simulink model "state_estimator"  (Simulink 9.1)
settings: Solver=VariableStepAuto  StartTime=0.0  StopTime=10.0  RelTol=1e-3
values from neighbouring files (symbols this model uses):
  Estimator =     [data_set.mat]
  g = 9.81    [data_set.mat]
  init =     [data_set.mat]
  Sensors =     [data_set.mat]
  Ts = 0.005    [data_set.mat]
undefined symbols (not defined in the file or in its folder): DiscIntNeverNeededParam, Discrete, Time
libraries: F_Line_block x281, simulink x27, ctrlSharedLib x3, sharedtransform x3, sharedutil x1
(part 1 of 2)
settings Model: LogicAnalyzerSignalOrdering=8909f14e-64a4-4a01-80b1-dba654a4ac6a  Creator=dongw  LastModifiedBy=dongw
settings DataIOCC: SaveFormat=Dataset
settings OptimizationCC: LifeSpan=auto
settings DebuggingCC: UnderspecifiedInitializationDetection=Simplified  MergeDetectMultiDrivingBlocksExec=error  SFUnexpectedBacktrackingDiag=error  SFNoUnconditionalDefaultTransitionDiag=error  SFExecutionAtInitializationDiag=warning
settings HardwareCC: ProdBitPerPointer=64  ProdBitPerSizeT=64  ProdBitPerPtrDiffT=64  ProdLargestAtomicFloat=Float  ProdIntDivRoundTo=Zero  ProdEndianess=LittleEndian  ProdWordSize=64  ProdHWDeviceType=Intel->x86-64 (Windows64)
settings ModelReferenceCC: PropagateSignalLabelsOutOfModel=on
settings CodeAppCC: StateflowObjectComments=off
settings GRTTargetCC: TargetLangStandard=C99 (ISO)  CombineOutputUpdateFcns=on  GRTInterface=off
settings ConfigComp: CovMetricSettings=dwe  CovHtmlReporting=off  CovSaveCumulativeToWorkspaceVar=off  CovSaveSingleToWorkspaceVar=off  CovExternalEMLEnable=on

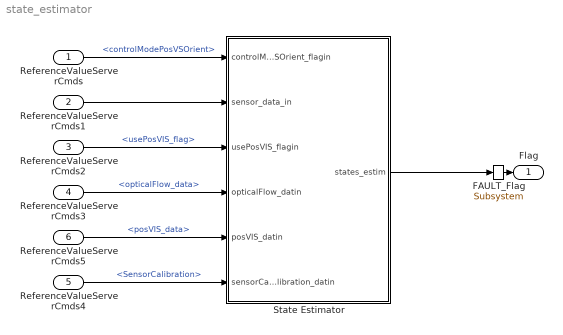
== system state_estimator ==
  ReferenceValueServerCmds : Inport  OutDataTypeStr=Bus: CommandBus
  ReferenceValueServerCmds1 : Inport  Port=2  OutDataTypeStr=Bus: CommandBus
  ReferenceValueServerCmds2 : Inport  Port=3  OutDataTypeStr=Bus: CommandBus
  ReferenceValueServerCmds3 : Inport  Port=4  OutDataTypeStr=Bus: CommandBus
  ReferenceValueServerCmds4 : Inport  Port=5  OutDataTypeStr=Bus: CommandBus
  ReferenceValueServerCmds5 : Inport  Port=6  OutDataTypeStr=Bus: CommandBus
  State Estimator : Subsystem
  Flag : Outport
  FAULT_Flag : F_Line_block/Subsystem
  wires:
  ReferenceValueServerCmds5/1 -> State Estimator/5(posVIS_datin)  "<posVIS_data>"
  State Estimator/1(states_estim) -> FAULT_Flag/1
  FAULT_Flag/1 -> Flag/1
  ReferenceValueServerCmds4/1 -> State Estimator/6(sensorCalibration_datin)  "<SensorCalibration>"
  ReferenceValueServerCmds2/1 -> State Estimator/3(usePosVIS_flagin)  "<usePosVIS_flag>"
  ReferenceValueServerCmds/1 -> State Estimator/1(controlModePosVSOrient_flagin)  "<controlModePosVSOrient>"
  ReferenceValueServerCmds3/1 -> State Estimator/4(opticalFlow_datin)  "<opticalFlow_data>"
  ReferenceValueServerCmds1/1 -> State Estimator/2(sensor_data_in)

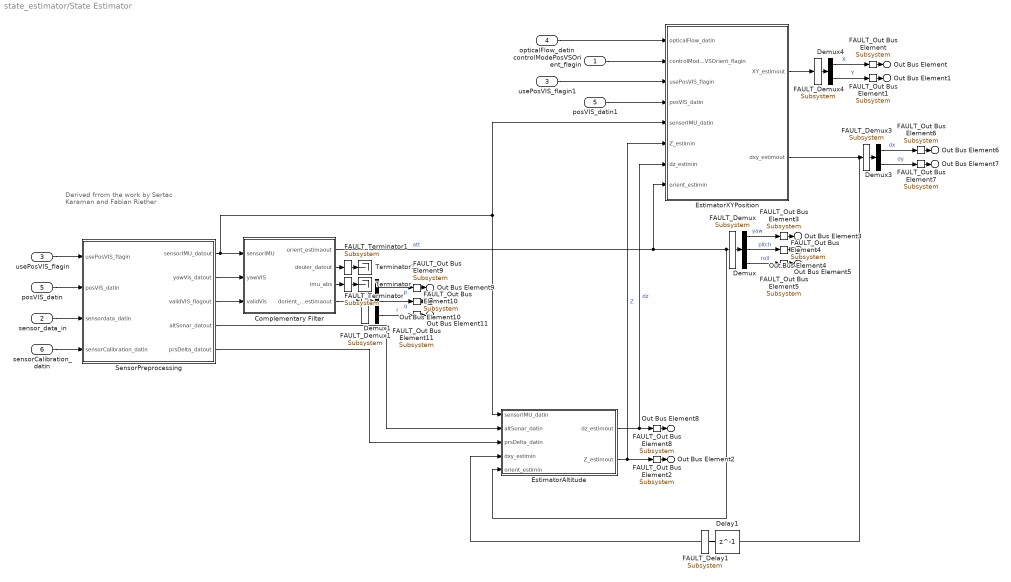
== system state_estimator/State Estimator ==
  note: Derived frrom the work by Sertac
      | Karaman and Fabian Riether
  controlModePosVSOrient_flagin : Inport  OutDataTypeStr=boolean
  sensor_data_in : Inport  Port=2
  usePosVIS_flagin : Inport  Port=3
  opticalFlow_datin : Inport  Port=4
  posVIS_datin : Inport  Port=5
  sensorCalibration_datin : Inport  Port=6
  Complementary Filter : Subsystem
  Delay1 : Delay  DelayLength=1  InitialCondition=0
  FAULT_Delay1 : F_Line_block/Subsystem
  Demux : Demux  Outputs=3
  FAULT_Demux{,1,3..4} (4 alike) : F_Line_block/Subsystem
  Demux1 : Demux  Outputs=3
  Demux3 : Demux  Outputs=2
  Demux4 : Demux  Outputs=2
  EstimatorAltitude : Subsystem
  EstimatorXYPosition : Subsystem
  SensorPreprocessing : Subsystem
  Terminator : Terminator
  FAULT_Terminator : F_Line_block/Subsystem
  Terminator1 : Terminator
  FAULT_Terminator1 : F_Line_block/Subsystem
  posVIS_datin1 : InportShadow  Port=5
  usePosVIS_flagin1 : InportShadow  Port=3
  Out Bus Element : Outport  PortName=states_estim  Element=X
  FAULT_Out Bus Element{,1..11} (12 alike) : F_Line_block/Subsystem
  Out Bus Element1 : Outport  PortName=states_estim  Element=Y
  Out Bus Element2 : Outport  PortName=states_estim  Element=Z
  Out Bus Element3 : Outport  PortName=states_estim  Element=yaw
  Out Bus Element4 : Outport  PortName=states_estim  Element=pitch
  Out Bus Element5 : Outport  PortName=states_estim  Element=roll
  Out Bus Element6 : Outport  PortName=states_estim  Element=dx
  Out Bus Element7 : Outport  PortName=states_estim  Element=dy
  Out Bus Element8 : Outport  PortName=states_estim  Element=dz
  Out Bus Element9 : Outport  PortName=states_estim  Element=p
  Out Bus Element10 : Outport  PortName=states_estim  Element=q
  Out Bus Element11 : Outport  PortName=states_estim  Element=r
  wires:
  EstimatorXYPosition/2(dxy_estimout) -> FAULT_Delay1/1, FAULT_Demux3/1
  ?FAULT_dxy_estimout_		DstPort			1/1 -> ?dxy_estimout/dstport			1
  ?FAULT_KalmanFilter_posxy/1 -> ?KalmanFilter_posxy/1
  ?FAULT_Mux1_6/1 -> ?Mux1/6
  ?FAULT_Product_2/1 -> ?Product/2
  FAULT_Delay1/1 -> Delay1/1
  FAULT_Demux3/1 -> Demux3/1
  posVIS_datin/1 -> SensorPreprocessing/2(posVIS_datin)
  Demux1/3 -> FAULT_Out Bus Element11/1  "r"
  FAULT_Out Bus Element11/1 -> Out Bus Element11/1
  Demux/3 -> FAULT_Out Bus Element5/1  "roll"
  FAULT_Out Bus Element5/1 -> Out Bus Element5/1
  Demux4/2 -> FAULT_Out Bus Element1/1  "Y"
  FAULT_Out Bus Element1/1 -> Out Bus Element1/1
  EstimatorXYPosition/1(XY_estimout) -> FAULT_Demux4/1
  FAULT_Demux4/1 -> Demux4/1
  Complementary Filter/2(deuler_datout) -> FAULT_Terminator1/1
  FAULT_Terminator1/1 -> Terminator1/1
  Complementary Filter/4(dorient_estimaout) -> FAULT_Demux1/1
  FAULT_Demux1/1 -> Demux1/1
  SensorPreprocessing/3(validVIS_flagout) -> Complementary Filter/3(validVis)
  sensor_data_in/1 -> SensorPreprocessing/3(sensordata_datin)
  opticalFlow_datin/1 -> EstimatorXYPosition/1(opticalFlow_datin)
  Demux4/1 -> FAULT_Out Bus Element/1  "X"
  FAULT_Out Bus Element/1 -> Out Bus Element/1
  SensorPreprocessing/1(sensorIMU_datout) -> Complementary Filter/1(sensorIMU), EstimatorAltitude/1(sensorIMU_datin), EstimatorXYPosition/5(sensorIMU_datin)
  SensorPreprocessing/5(prsDelta_datout) -> EstimatorAltitude/3(prsDelta_datin)
  Demux3/2 -> FAULT_Out Bus Element7/1  "dy"
  ?FAULT_dxy_estimout_		DstPort			1/1 -> ?dxy_estimout/dstport			1
  ?FAULT_KalmanFilter_posxy/1 -> ?KalmanFilter_posxy/1
  ?FAULT_Mux1_6/1 -> ?Mux1/6
  FAULT_Out Bus Element7/1 -> Out Bus Element7/1
  SensorPreprocessing/2(yawVis_datout) -> Complementary Filter/2(yawVIS)
  SensorPreprocessing/4(altSonar_datout) -> EstimatorAltitude/2(altSonar_datin)
  usePosVIS_flagin/1 -> SensorPreprocessing/1(usePosVIS_flagin)
  EstimatorAltitude/1(dz_estimout) -> FAULT_Out Bus Element8/1, EstimatorXYPosition/7(dz_estimin)  "dz"
  FAULT_Out Bus Element8/1 -> Out Bus Element8/1
  ?FAULT_KalmanFilter_posxy/1 -> ?KalmanFilter_posxy/1
  EstimatorAltitude/2(Z_estimout) -> FAULT_Out Bus Element2/1, EstimatorXYPosition/6(Z_estimin)  "Z"
  FAULT_Out Bus Element2/1 -> Out Bus Element2/1
  ?FAULT_KalmanFilter_posxy/1 -> ?KalmanFilter_posxy/1
  Demux1/1 -> FAULT_Out Bus Element9/1  "p"
  FAULT_Out Bus Element9/1 -> Out Bus Element9/1
  Demux3/1 -> FAULT_Out Bus Element6/1  "dx"
  FAULT_Out Bus Element6/1 -> Out Bus Element6/1
  Complementary Filter/3(imu_abs) -> FAULT_Terminator/1
  FAULT_Terminator/1 -> Terminator/1
  Demux/2 -> FAULT_Out Bus Element4/1  "pitch"
  FAULT_Out Bus Element4/1 -> Out Bus Element4/1
  controlModePosVSOrient_flagin/1 -> EstimatorXYPosition/2(controlModePosVSOrient_flagin)
  Complementary Filter/1(orient_estimaout) -> EstimatorAltitude/5(orient_estimin), Demux/1, EstimatorXYPosition/8(orient_estimin)  "att"
  Demux/1 -> FAULT_Out Bus Element3/1  "yaw"
  FAULT_Out Bus Element2/1 -> Out Bus Element2/1
  FAULT_Out Bus Element3/1 -> Out Bus Element3/1
  Delay1/1 -> EstimatorAltitude/4(dxy_estimin)
  Demux1/2 -> FAULT_Out Bus Element10/1  "q"
  FAULT_Out Bus Element10/1 -> Out Bus Element10/1
  usePosVIS_flagin1/1 -> EstimatorXYPosition/3(usePosVIS_flagin)
  posVIS_datin1/1 -> EstimatorXYPosition/4(posVIS_datin)
  sensorCalibration_datin/1 -> SensorPreprocessing/4(sensorCalibration_datin)

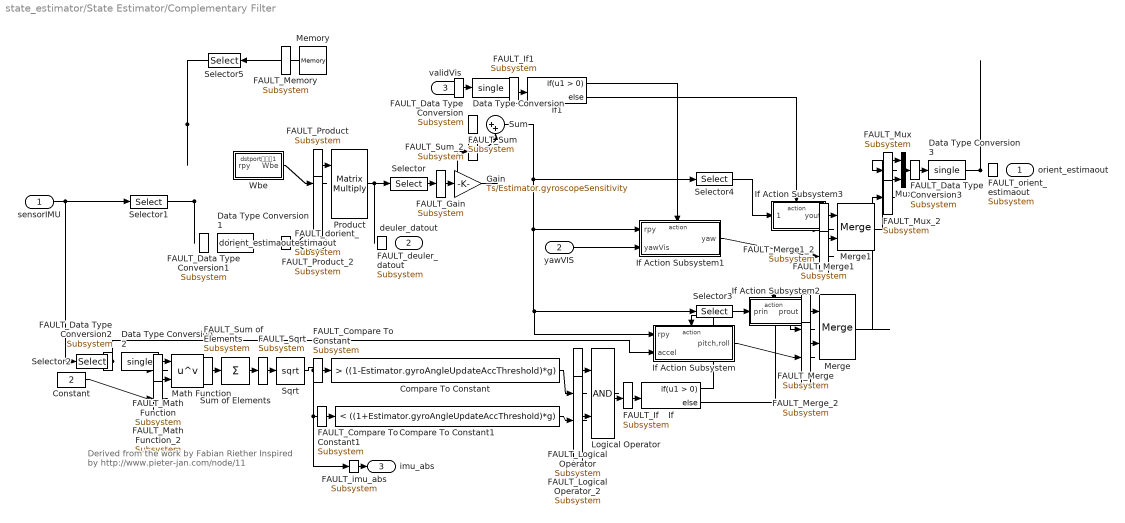
== system state_estimator/State Estimator/Complementary Filter ==
  note: Derived from the work by Fabian Riether
      | Inspired by http://www.pieter-jan.com/node/11
  sensorIMU : Inport  OutDataTypeStr=single
  yawVIS : Inport  Port=2
  validVis : Inport  Port=3
  Compare To Constant : simulink/Logic and Bit Operations/Compare To Constant  relop=>  const=((1-Estimator.gyroAngleUpdateAccThreshold)*g)  OutDataTypeStr=boolean
  FAULT_Compare To Constant : F_Line_block/Subsystem
  Compare To Constant1 : simulink/Logic and Bit Operations/Compare To Constant  relop=<  const=((1+Estimator.gyroAngleUpdateAccThreshold)*g)  OutDataTypeStr=boolean
  FAULT_Compare To Constant1 : F_Line_block/Subsystem
  Constant : Constant  Value=2  OutDataTypeStr=single
  Data Type Conversion{,1..3} (4 alike) : DataTypeConversion  OutDataTypeStr=single
  FAULT_Data Type Conversion{,1..3} (4 alike) : F_Line_block/Subsystem
  Gain : Gain  Gain=Ts/Estimator.gyroscopeSensitivity
  FAULT_Gain : F_Line_block/Subsystem
  If : If
  FAULT_If : F_Line_block/Subsystem
  If Action Subsystem : Subsystem  TreatAsAtomicUnit=on
  If Action Subsystem1 : Subsystem  TreatAsAtomicUnit=on
  If Action Subsystem2 : Subsystem  TreatAsAtomicUnit=on
  If Action Subsystem3 : Subsystem  TreatAsAtomicUnit=on
  If1 : If
  FAULT_If1 : F_Line_block/Subsystem
  Logical Operator : Logic  AllPortsSameDT=off  OutDataTypeStr=fixdt(1,16)
  FAULT_Logical Operator : F_Line_block/Subsystem
  FAULT_Logical Operator_2 : F_Line_block/Subsystem
  Math Function : Math  Operator=pow  SaturateOnIntegerOverflow=on
  FAULT_Math Function : F_Line_block/Subsystem
  FAULT_Math Function_2 : F_Line_block/Subsystem
  Memory : Memory  InitialCondition=single(Estimator.complementaryFilterInit)  InheritSampleTime=on
  FAULT_Memory : F_Line_block/Subsystem
  Merge : Merge
  FAULT_Merge : F_Line_block/Subsystem
  FAULT_Merge_2 : F_Line_block/Subsystem
  Merge1 : Merge
  FAULT_Merge1 : F_Line_block/Subsystem
  FAULT_Merge1_2 : F_Line_block/Subsystem
  Mux : Mux  Inputs=2
  FAULT_Mux : F_Line_block/Subsystem
  FAULT_Mux_2 : F_Line_block/Subsystem
  Product : Product  Multiplication=Matrix(*)
  FAULT_Product : F_Line_block/Subsystem
  FAULT_Product_2 : F_Line_block/Subsystem
  Selector : Selector  InputPortWidth=3  IndexOptions=Index vector (dialog)  Indices=[3 2 1]  OutputSizes=1
  Selector1 : Selector  InputPortWidth=6  IndexOptions=Index vector (dialog)  Indices=[4 5 6]  OutputSizes=1
  Selector2 : Selector  InputPortWidth=6  IndexOptions=Index vector (dialog)  Indices=[1 2 3]  OutputSizes=1
  Selector3 : Selector  InputPortWidth=3  IndexOptions=Index vector (dialog)  Indices=[2 1]  OutputSizes=1
  Selector4 : Selector  InputPortWidth=3  IndexOptions=Index vector (dialog)  Indices=[3]  OutputSizes=1
  Selector5 : Selector  InputPortWidth=3  IndexOptions=Index vector (dialog)  Indices=[3 2 1]  OutputSizes=1
  Sqrt : Sqrt  SaturateOnIntegerOverflow=on
  FAULT_Sqrt : F_Line_block/Subsystem
  Sum : Sum  Inputs=|++
  FAULT_Sum : F_Line_block/Subsystem
  FAULT_Sum_2 : F_Line_block/Subsystem
  Sum of Elements : Sum  Inputs=+
  FAULT_Sum of Elements : F_Line_block/Subsystem
  Wbe : Subsystem
  orient_estimaout : Outport
  FAULT_orient_estimaout : F_Line_block/Subsystem
  deuler_datout : Outport  Port=2
  FAULT_deuler_datout : F_Line_block/Subsystem
  imu_abs : Outport  Port=3  OutDataTypeStr=single
  FAULT_imu_abs : F_Line_block/Subsystem
  dorient_estimaout : Outport  Port=4
  FAULT_dorient_estimaout : F_Line_block/Subsystem
  wires:
  sensorIMU/1 -> Selector1/1, Selector2/1
  Product/1 -> ?FAULT_deuler_datout_		DstPort			1/1, Selector/1
  ?FAULT_Product3/1 -> ?Product3/1
  ?FAULT_Create 3x3 Matrix/1 -> ?Create 3x3 Matrix/1
  ?FAULT_deuler_datout_		DstPort			1/1 -> deuler_datout/dstport			1
  ?FAULT_Product3_2/1 -> ?Product3/2
  Wbe/1(Wbe) -> FAULT_Product/1
  FAULT_Product/1 -> Product/1
  Selector/1 -> FAULT_Gain/1
  FAULT_Gain/1 -> Gain/1
  Gain/1 -> FAULT_Sum_2/1
  FAULT_Sum_2/1 -> Sum/2
  Memory/1 -> Selector5/1
  Sum of Elements/1 -> FAULT_Sqrt/1
  FAULT_Sqrt/1 -> Sqrt/1
  Math Function/1 -> FAULT_Sum of Elements/1
  FAULT_Sum of Elements/1 -> Sum of Elements/1
  Constant/1 -> FAULT_Math Function_2/1
  FAULT_Math Function_2/1 -> Math Function/2
  Selector2/1 -> If Action Subsystem/2(accel), ?FAULT_Data Type Conversion2_		DstPort			1/1
  ?FAULT_Product3/1 -> ?Product3/1
  ?FAULT_Data Type Conversion2_		DstPort			1/1 -> Data Type Conversion2/dstport			1
  Sqrt/1 -> FAULT_imu_abs/1, Compare To Constant1/1, Compare To Constant/1
  Compare To Constant/1 -> FAULT_Logical Operator/1
  FAULT_Logical Operator/1 -> Logical Operator/1
  Compare To Constant1/1 -> FAULT_Logical Operator_2/1
  FAULT_Logical Operator_2/1 -> Logical Operator/2
  If Action Subsystem/1(pitch,roll) -> FAULT_Merge_2/1
  FAULT_Merge_2/1 -> Merge/2
  Sum/1 -> If Action Subsystem1/1(rpy), If Action Subsystem/1(rpy), Selector3/1, Selector4/1
  Selector3/1 -> If Action Subsystem2/1(prin)
  yawVIS/1 -> If Action Subsystem1/2(yawVis)
  Selector4/1 -> If Action Subsystem3/1(yawin)
  If Action Subsystem1/1(yaw) -> FAULT_Merge1_2/1
  FAULT_imu_abs/1 -> imu_abs/1
  ?FAULT_Data Type Conversion2_		DstPort			1/1 -> Data Type Conversion2/dstport			1
  ?FAULT_deuler_datout_		DstPort			1/1 -> deuler_datout/dstport			1
  ?FAULT_Product3_2/1 -> ?Product3/2
  FAULT_Merge1_2/1 -> Merge1/2
  Merge/1 -> FAULT_Mux_2/1
  FAULT_Mux_2/1 -> Mux/2
  Mux/1 -> FAULT_Data Type Conversion3/1
  FAULT_Data Type Conversion3/1 -> Data Type Conversion3/1
  If Action Subsystem2/1(prout) -> FAULT_Merge/1
  FAULT_Merge/1 -> Merge/1
  If/2 -> If Action Subsystem2/Action
  If Action Subsystem3/1(yout) -> FAULT_Merge1/1
  FAULT_Merge1/1 -> Merge1/1
  If1/2 -> If Action Subsystem3/Action
  Logical Operator/1 -> FAULT_If/1
  FAULT_If/1 -> If/1
  If/1 -> If Action Subsystem/Action
  If1/1 -> If Action Subsystem1/Action
  Data Type Conversion/1 -> FAULT_If1/1
  FAULT_If1/1 -> If1/1
  validVis/1 -> FAULT_Data Type Conversion/1
  FAULT_Data Type Conversion/1 -> Data Type Conversion/1
  Selector1/1 -> ?FAULT_Product_		DstPort			2/1, ?FAULT_Data Type Conversion1_		DstPort			1/1
  ?FAULT_Product_		DstPort			2/1 -> Product/dstport			2
  ?FAULT_Data Type Conversion1_		DstPort			1/1 -> Data Type Conversion1/dstport			1
  Data Type Conversion2/1 -> FAULT_Math Function/1
  FAULT_Math Function/1 -> Math Function/1
  Data Type Conversion3/1 -> ?FAULT_Memory_		DstPort			1/1, ?FAULT_orient_estimaout_		DstPort			1/1
  ?FAULT_Memory_		DstPort			1/1 -> Memory/dstport			1
  ?FAULT_orient_estimaout_		DstPort			1/1 -> orient_estimaout/dstport			1
  Merge1/1 -> FAULT_Mux/1
  FAULT_Mux/1 -> Mux/1
  Selector5/1 -> ?FAULT_Sum_		DstPort			1/1, ?FAULT_Wbe_		DstPort			1/1
  ?FAULT_Sum_		DstPort			1/1 -> Sum/dstport			1
  ?FAULT_Wbe_		DstPort			1/1 -> Wbe/dstport			1
  Data Type Conversion1/1 -> FAULT_dorient_estimaout/1
  FAULT_dorient_estimaout/1 -> dorient_estimaout/1

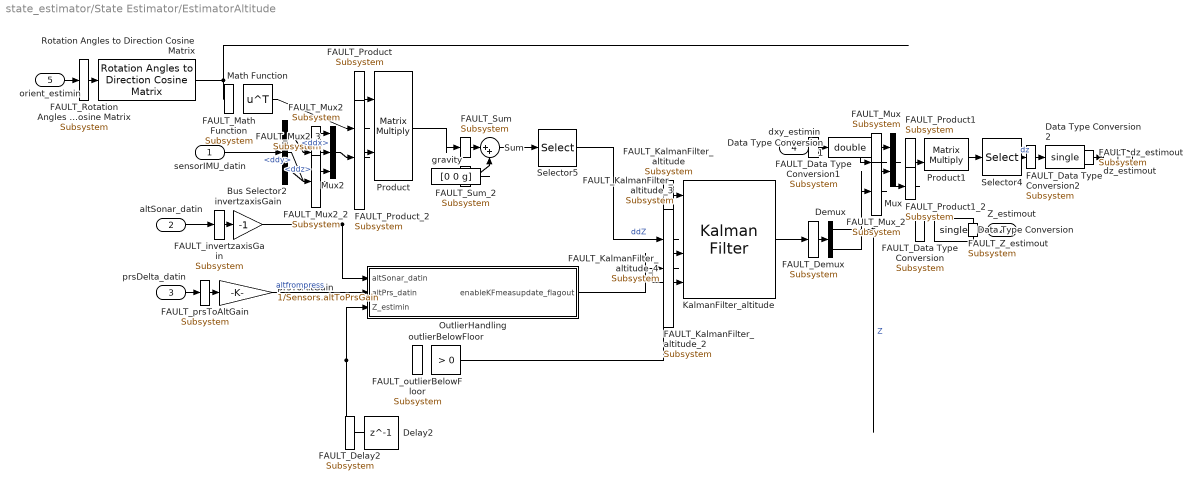
== system state_estimator/State Estimator/EstimatorAltitude ==
  sensorIMU_datin : Inport
  altSonar_datin : Inport  Port=2
  prsDelta_datin : Inport  Port=3
  dxy_estimin : Inport  Port=4
  orient_estimin : Inport  Port=5
  Bus Selector2 : BusSelector  OutputSignals=ddx,ddy,ddz
  Data Type Conversion : DataTypeConversion  OutDataTypeStr=single  SaturateOnIntegerOverflow=on
  FAULT_Data Type Conversion : F_Line_block/Subsystem
  Data Type Conversion1 : DataTypeConversion  OutDataTypeStr=double  SaturateOnIntegerOverflow=on
  FAULT_Data Type Conversion1 : F_Line_block/Subsystem
  Data Type Conversion2 : DataTypeConversion  OutDataTypeStr=single  SaturateOnIntegerOverflow=on
  FAULT_Data Type Conversion2 : F_Line_block/Subsystem
  Delay2 : Delay  DelayLength=1  InitialCondition=0
  FAULT_Delay2 : F_Line_block/Subsystem
  Demux : Demux  Outputs=2
  FAULT_Demux : F_Line_block/Subsystem
  KalmanFilter_altitude : ctrlSharedLib/Kalman Filter  TimeDomain=Discrete-Time  UseCurrentEstimator=on  ModelSource=Individual A, B, C, D matrices  ModelSourceVariable=sys  A=[1 Ts; 0 1]  B=[0;Ts]  C=[1 0]  D=[0]  NumberOfStates=2  NumberOfInputs=2  NumberOfOutputs=2  InitialEstimateSource=Dialog  X0=[init.posNED(3) 0]  P0=10  UseK=off  UseGH=on  NumberOfProcessNoiseInputs=2  G=Estimator.alt.kf.G  TimeInvariantG=on  H=Estimator.alt.kf.H  TimeInvariantH=on  Q=Estimator.alt.kf.Q  TimeInvariantQ=on  R=Estimator.alt.kf.R  TimeInvariantR=on  N=Estimator.alt.kf.N  TimeInvariantN=on  AddInputPort=on  AddEnablePort=on  ExternalReset=Level hold  OutputEstimatedY=off  OutputP=off  Ts=-1
      settings: SourceProductBaseCode=CT
  FAULT_KalmanFilter_altitude : F_Line_block/Subsystem
  FAULT_KalmanFilter_altitude_2 : F_Line_block/Subsystem
  FAULT_KalmanFilter_altitude_3 : F_Line_block/Subsystem
  FAULT_KalmanFilter_altitude_4 : F_Line_block/Subsystem
  Math Function : Math  Operator=transpose  SaturateOnIntegerOverflow=on
  FAULT_Math Function : F_Line_block/Subsystem
  Mux : Mux  Inputs=2
  FAULT_Mux : F_Line_block/Subsystem
  FAULT_Mux_2 : F_Line_block/Subsystem
  Mux2 : Mux  Inputs=3
  FAULT_Mux2 : F_Line_block/Subsystem
  FAULT_Mux2_2 : F_Line_block/Subsystem
  FAULT_Mux2_3 : F_Line_block/Subsystem
  OutlierHandling : Subsystem
  Product : Product  Multiplication=Matrix(*)
  FAULT_Product : F_Line_block/Subsystem
  FAULT_Product_2 : F_Line_block/Subsystem
  Product1 : Product  Multiplication=Matrix(*)
  FAULT_Product1 : F_Line_block/Subsystem
  FAULT_Product1_2 : F_Line_block/Subsystem
  Rotation Angles to Direction Cosine Matrix : sharedtransform/Rotation Angles to Direction Cosine Matrix  rotationOrder=ZYX  aMode=aMode
      settings: SourceProductBaseCode=AE
  FAULT_Rotation Angles to Direction Cosine Matrix : F_Line_block/Subsystem
  Selector4 : Selector  InputPortWidth=3  IndexOptions=Index vector (dialog)  Indices=[3]  OutputSizes=1
  Selector5 : Selector  InputPortWidth=3  IndexOptions=Index vector (dialog)  Indices=[3]  OutputSizes=1
  Sum : Sum  Inputs=|++
  FAULT_Sum : F_Line_block/Subsystem
  FAULT_Sum_2 : F_Line_block/Subsystem
  gravity : Constant  Value=[0 0 g]
  invertzaxisGain : Gain  Gain=-1  ParamDataTypeStr=single  OutDataTypeStr=double
  FAULT_invertzaxisGain : F_Line_block/Subsystem
  outlierBelowFloor : simulink/Logic and Bit Operations/Compare To Constant  relop=>  const=0  OutDataTypeStr=boolean
  FAULT_outlierBelowFloor : F_Line_block/Subsystem
  prsToAltGain : Gain  Gain=1/Sensors.altToPrsGain
  FAULT_prsToAltGain : F_Line_block/Subsystem
  dz_estimout : Outport
  FAULT_dz_estimout : F_Line_block/Subsystem
  Z_estimout : Outport  Port=2
  FAULT_Z_estimout : F_Line_block/Subsystem
  wires:
  Mux2/1 -> FAULT_Product_2/1
  FAULT_Product_2/1 -> Product/2
  sensorIMU_datin/1 -> Bus Selector2/1
  Bus Selector2/3 -> FAULT_Mux2_3/1  "<ddz>"
  FAULT_Mux2_3/1 -> Mux2/3
  Bus Selector2/2 -> FAULT_Mux2_2/1  "<ddy>"
  FAULT_Mux2_2/1 -> Mux2/2
  Bus Selector2/1 -> FAULT_Mux2/1  "<ddx>"
  FAULT_Mux2/1 -> Mux2/1
  Product1/1 -> Selector4/1
  dxy_estimin/1 -> FAULT_Data Type Conversion1/1
  FAULT_Data Type Conversion1/1 -> Data Type Conversion1/1
  Delay2/1 -> OutlierHandling/3(Z_estimin), ?FAULT_outlierBelowFloor_		DstPort			1/1
  ?FAULT_Add1/1 -> ?Add1/1
  ?FAULT_outlierBelowFloor_		DstPort			1/1 -> outlierBelowFloor/dstport			1
  prsToAltGain/1 -> OutlierHandling/2(altPrs_datin)  "altfrompress"
  prsDelta_datin/1 -> FAULT_prsToAltGain/1
  FAULT_prsToAltGain/1 -> prsToAltGain/1
  outlierBelowFloor/1 -> FAULT_KalmanFilter_altitude_4/1
  FAULT_KalmanFilter_altitude_4/1 -> KalmanFilter_altitude/4
  Demux/2 -> FAULT_Mux_2/1
  FAULT_Mux_2/1 -> Mux/2
  Selector4/1 -> FAULT_Data Type Conversion2/1  "dz"
  FAULT_Data Type Conversion2/1 -> Data Type Conversion2/1
  Demux/1 -> ?FAULT_Data Type Conversion_		DstPort			1/1, ?FAULT_Delay2_		DstPort			1/1  "Z"
  ?FAULT_Data Type Conversion_		DstPort			1/1 -> Data Type Conversion/dstport			1
  ?FAULT_Delay2_		DstPort			1/1 -> Delay2/dstport			1
  Selector5/1 -> FAULT_KalmanFilter_altitude/1  "ddZ"
  FAULT_KalmanFilter_altitude/1 -> KalmanFilter_altitude/1
  Mux/1 -> FAULT_Product1_2/1
  FAULT_Product1_2/1 -> Product1/2
  KalmanFilter_altitude/1 -> FAULT_Demux/1
  FAULT_Demux/1 -> Demux/1
  Sum/1 -> Selector5/1
  gravity/1 -> FAULT_Sum_2/1
  FAULT_Sum_2/1 -> Sum/2
  Product/1 -> FAULT_Sum/1
  FAULT_Sum/1 -> Sum/1
  altSonar_datin/1 -> FAULT_invertzaxisGain/1
  FAULT_invertzaxisGain/1 -> invertzaxisGain/1
  orient_estimin/1 -> FAULT_Rotation Angles to Direction Cosine Matrix/1
  FAULT_Rotation Angles to Direction Cosine Matrix/1 -> Rotation Angles to Direction Cosine Matrix/1
  Data Type Conversion/1 -> FAULT_Z_estimout/1
  FAULT_Z_estimout/1 -> Z_estimout/1
  Data Type Conversion1/1 -> FAULT_Mux/1
  FAULT_Mux/1 -> Mux/1
  Math Function/1 -> FAULT_Product/1
  FAULT_Product/1 -> Product/1
  invertzaxisGain/1 -> ?FAULT_KalmanFilter_altitude_		DstPort			2/1, OutlierHandling/1(altSonar_datin)
  ?FAULT_KalmanFilter_altitude_		DstPort			2/1 -> KalmanFilter_altitude/dstport			2
  ?FAULT_Delay2_		DstPort			1/1 -> Delay2/dstport			1
  Data Type Conversion2/1 -> FAULT_dz_estimout/1
  FAULT_dz_estimout/1 -> dz_estimout/1
  OutlierHandling/1(enableKFmeasupdate_flagout) -> FAULT_KalmanFilter_altitude_3/1
  FAULT_KalmanFilter_altitude_3/1 -> KalmanFilter_altitude/3
  Rotation Angles to Direction Cosine Matrix/1 -> ?FAULT_Math Function_		DstPort			1/1, ?FAULT_Product1_		DstPort			1/1
  ?FAULT_Math Function_		DstPort			1/1 -> Math Function/dstport			1
  ?FAULT_Product1_		DstPort			1/1 -> Product1/dstport			1

== system state_estimator/State Estimator/EstimatorXYPosition ==
  opticalFlow_datin : Inport
  controlModePosVSOrient_flagin : Inport  Port=2
  usePosVIS_flagin : Inport  Port=3
  posVIS_datin : Inport  Port=4
  sensorIMU_datin : Inport  Port=5
  Z_estimin : Inport  Port=6
  dz_estimin : Inport  Port=7
  orient_estimin : Inport  Port=8
  EstimatorVelocity : Subsystem
  EstimatorXYPosition : Subsystem
  XY_estimout : Outport
  FAULT_XY_estimout : F_Line_block/Subsystem
  dxy_estimout : Outport  Port=2
  FAULT_dxy_estimout : F_Line_block/Subsystem
  wires:
  EstimatorXYPosition/1(XY_estimout) -> FAULT_XY_estimout/1
  FAULT_XY_estimout/1 -> XY_estimout/1
  usePosVIS_flagin/1 -> EstimatorXYPosition/6(usePosVIS_flagin)
  posVIS_datin/1 -> EstimatorXYPosition/5(posVIS_datin)
  dz_estimin/1 -> EstimatorXYPosition/4(dz_estimin)
  controlModePosVSOrient_flagin/1 -> EstimatorXYPosition/3(controlModePosVSOrient_flagin)
  Z_estimin/1 -> EstimatorVelocity/2(Z_estimin)
  sensorIMU_datin/1 -> EstimatorVelocity/3(sensorIMU_datin)
  opticalFlow_datin/1 -> EstimatorVelocity/1(opticalFlow_datin)
  EstimatorVelocity/1(dxy_estimout) -> ?FAULT_dxy_estimout_		DstPort			1/1, EstimatorXYPosition/1(dxy_estimin)
  ?FAULT_dxy_estimout_		DstPort			1/1 -> dxy_estimout/dstport			1
  ?FAULT_KalmanFilter_posxy/1 -> ?KalmanFilter_posxy/1
  orient_estimin/1 -> EstimatorXYPosition/2(orient_estimin), EstimatorVelocity/4(orient_estimin)

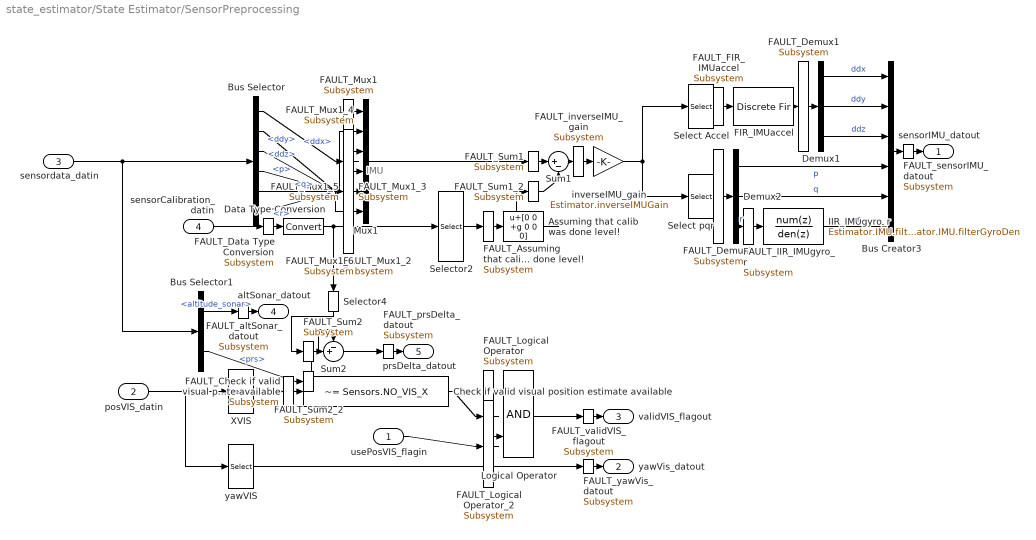
== system state_estimator/State Estimator/SensorPreprocessing ==
  note: IMU
  usePosVIS_flagin : Inport
  posVIS_datin : Inport  Port=2
  sensordata_datin : Inport  Port=3
  sensorCalibration_datin : Inport  Port=4
  Assuming that calib was done level! : Bias  Bias=[0 0 +g 0 0 0]
  FAULT_Assuming that calib was done level! : F_Line_block/Subsystem
  Bus Creator3 : BusCreator  Inputs=6
  Bus Selector : BusSelector  OutputSignals=ddx,ddy,ddz,p,q,r
  Bus Selector1 : BusSelector  OutputSignals=altitude_sonar,prs
  Check if valid visual position estimate available : simulink/Logic and Bit Operations/Compare To Constant  relop=~=  const=Sensors.NO_VIS_X  OutDataTypeStr=boolean
  FAULT_Check if valid visual position estimate available : F_Line_block/Subsystem
  Data Type Conversion : DataTypeConversion
  FAULT_Data Type Conversion : F_Line_block/Subsystem
  Demux1 : Demux  Outputs=3
  FAULT_Demux1 : F_Line_block/Subsystem
  Demux2 : Demux  Outputs=3
  FAULT_Demux2 : F_Line_block/Subsystem
  FIR_IMUaccel : DiscreteFir  Coefficients=Estimator.IMU.filterAccel.Coefficients
  FAULT_FIR_IMUaccel : F_Line_block/Subsystem
  IIR_IMUgyro_r : DiscreteFilter  Numerator=Estimator.IMU.filterGyroNum  Denominator=Estimator.IMU.filterGyroDen
  FAULT_IIR_IMUgyro_r : F_Line_block/Subsystem
  Logical Operator : Logic  AllPortsSameDT=off  OutDataTypeStr=boolean
  FAULT_Logical Operator : F_Line_block/Subsystem
  FAULT_Logical Operator_2 : F_Line_block/Subsystem
  Mux1 : Mux  Inputs=6
  FAULT_Mux1 : F_Line_block/Subsystem
  FAULT_Mux1_{2..6} (5 alike) : F_Line_block/Subsystem
  Select Accel : Selector  InputPortWidth=6  IndexOptions=Index vector (dialog)  Indices=[1 2 3]  OutputSizes=1
  Select pqr : Selector  InputPortWidth=6  IndexOptions=Index vector (dialog)  Indices=[4 5 6]  OutputSizes=1
  Selector2 : Selector  InputPortWidth=8  IndexOptions=Index vector (dialog)  Indices=[1:6]  OutputSizes=1
  Selector4 : Selector  InputPortWidth=8  IndexOptions=Index vector (dialog)  Indices=[7]  OutputSizes=1
  Sum1 : Sum  Inputs=|+-
  FAULT_Sum1 : F_Line_block/Subsystem
  FAULT_Sum1_2 : F_Line_block/Subsystem
  Sum2 : Sum  Inputs=-+|
  FAULT_Sum2 : F_Line_block/Subsystem
  FAULT_Sum2_2 : F_Line_block/Subsystem
  XVIS : Selector  InputPortWidth=4  IndexOptions=Index vector (dialog)  Indices=1  OutputSizes=1
  inverseIMU_gain : Gain  Gain=Estimator.inverseIMUGain  ParamDataTypeStr=single  OutDataTypeStr=single
  FAULT_inverseIMU_gain : F_Line_block/Subsystem
  yawVIS : Selector  InputPortWidth=4  IndexOptions=Index vector (dialog)  Indices=4  OutputSizes=1
  sensorIMU_datout : Outport
  FAULT_sensorIMU_datout : F_Line_block/Subsystem
  yawVis_datout : Outport  Port=2
  FAULT_yawVis_datout : F_Line_block/Subsystem
  validVIS_flagout : Outport  Port=3
  FAULT_validVIS_flagout : F_Line_block/Subsystem
  altSonar_datout : Outport  Port=4
  FAULT_altSonar_datout : F_Line_block/Subsystem
  prsDelta_datout : Outport  Port=5
  FAULT_prsDelta_datout : F_Line_block/Subsystem
  wires:
  Select pqr/1 -> FAULT_Demux2/1
  ?FAULT_dxy_estimout_		DstPort			1/1 -> ?dxy_estimout/dstport			1
  ?FAULT_KalmanFilter_posxy/1 -> ?KalmanFilter_posxy/1
  FAULT_Demux2/1 -> Demux2/1
  Assuming that calib was done level!/1 -> FAULT_Sum1_2/1
  FAULT_Sum1_2/1 -> Sum1/2
  usePosVIS_flagin/1 -> FAULT_Logical Operator_2/1
  FAULT_Logical Operator_2/1 -> Logical Operator/2
  Check if valid visual position estimate available/1 -> FAULT_Logical Operator/1
  FAULT_Logical Operator/1 -> Logical Operator/1
  Logical Operator/1 -> FAULT_validVIS_flagout/1
  FAULT_validVIS_flagout/1 -> validVIS_flagout/1
  yawVIS/1 -> FAULT_yawVis_datout/1
  FAULT_yawVis_datout/1 -> yawVis_datout/1
  XVIS/1 -> FAULT_Check if valid visual position estimate available/1
  FAULT_Check if valid visual position estimate available/1 -> Check if valid visual position estimate available/1
  Mux1/1 -> FAULT_Sum1/1
  FAULT_Sum1/1 -> Sum1/1
  Sum2/1 -> FAULT_prsDelta_datout/1
  FAULT_prsDelta_datout/1 -> prsDelta_datout/1
  Bus Selector1/2 -> FAULT_Sum2_2/1  "<prs>"
  FAULT_Sum2_2/1 -> Sum2/2
  Selector4/1 -> FAULT_Sum2/1
  FAULT_Sum2/1 -> Sum2/1
  Bus Selector1/1 -> FAULT_altSonar_datout/1  "<altitude_sonar>"
  FAULT_altSonar_datout/1 -> altSonar_datout/1
  sensordata_datin/1 -> Bus Selector1/1, Bus Selector/1
  Bus Selector/6 -> FAULT_Mux1_6/1  "<r>"
  ?FAULT_dxy_estimout_		DstPort			1/1 -> ?dxy_estimout/dstport			1
  ?FAULT_KalmanFilter_posxy/1 -> ?KalmanFilter_posxy/1
  FAULT_Mux1_6/1 -> Mux1/6
  Bus Selector/5 -> FAULT_Mux1_5/1  "<q>"
  FAULT_Mux1_5/1 -> Mux1/5
  Bus Selector/4 -> FAULT_Mux1_4/1  "<p>"
  FAULT_Mux1_4/1 -> Mux1/4
  Bus Selector/3 -> FAULT_Mux1_3/1  "<ddz>"
  FAULT_Mux1_3/1 -> Mux1/3
  Bus Selector/2 -> FAULT_Mux1_2/1  "<ddy>"
  FAULT_Mux1_2/1 -> Mux1/2
  Bus Selector/1 -> FAULT_Mux1/1  "<ddx>"
  FAULT_Mux1/1 -> Mux1/1
  sensorCalibration_datin/1 -> FAULT_Data Type Conversion/1
  FAULT_Data Type Conversion/1 -> Data Type Conversion/1
  IIR_IMUgyro_r/1 -> Bus Creator3/6  "r"
  Demux2/3 -> FAULT_IIR_IMUgyro_r/1  "r"
  FAULT_IIR_IMUgyro_r/1 -> IIR_IMUgyro_r/1
  FIR_IMUaccel/1 -> FAULT_Demux1/1
  FAULT_Demux1/1 -> Demux1/1
  Select Accel/1 -> FAULT_FIR_IMUaccel/1
  FAULT_FIR_IMUaccel/1 -> FIR_IMUaccel/1
  inverseIMU_gain/1 -> Select Accel/1, Select pqr/1
  Demux2/2 -> Bus Creator3/5  "q"
  Demux2/1 -> Bus Creator3/4  "p"
  Selector2/1 -> FAULT_Assuming that calib was done level!/1
  ?FAULT_dxy_estimout_		DstPort			1/1 -> ?dxy_estimout/dstport			1
  ?FAULT_KalmanFilter_posxy/1 -> ?KalmanFilter_posxy/1
  FAULT_Mux1_6/1 -> Mux1/6
  ?FAULT_Product_2/1 -> ?Product/2
  FAULT_Assuming that calib was done level!/1 -> Assuming that calib was done level!/1
  Sum1/1 -> FAULT_inverseIMU_gain/1
  FAULT_inverseIMU_gain/1 -> inverseIMU_gain/1
  Demux1/3 -> Bus Creator3/3  "ddz"
  Demux1/2 -> Bus Creator3/2  "ddy"
  Demux1/1 -> Bus Creator3/1  "ddx"
  Bus Creator3/1 -> FAULT_sensorIMU_datout/1
  FAULT_sensorIMU_datout/1 -> sensorIMU_datout/1
  posVIS_datin/1 -> XVIS/1, yawVIS/1
  Data Type Conversion/1 -> Selector2/1, Selector4/1

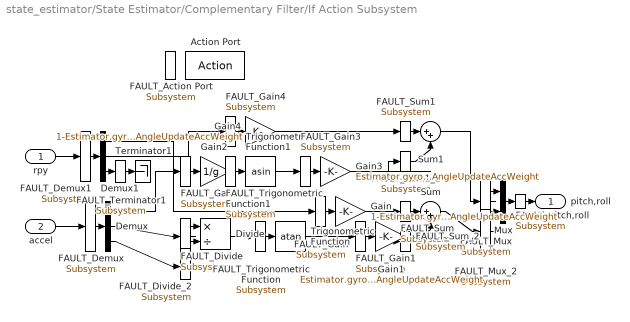
== system state_estimator/State Estimator/Complementary Filter/If Action Subsystem ==
  rpy : Inport
  accel : Inport  Port=2
  Action Port : ActionPort
  FAULT_Action Port : F_Line_block/Subsystem
  Demux : Demux  Outputs=3
  FAULT_Demux : F_Line_block/Subsystem
  Demux1 : Demux  Outputs=3
  FAULT_Demux1 : F_Line_block/Subsystem
  Divide : Product  Inputs=*/
  FAULT_Divide : F_Line_block/Subsystem
  FAULT_Divide_2 : F_Line_block/Subsystem
  Gain : Gain  Gain=1-Estimator.gyroAngleUpdateAccWeight
  FAULT_Gain{,1..4} (5 alike) : F_Line_block/Subsystem
  Gain1 : Gain  Gain=Estimator.gyroAngleUpdateAccWeight
  Gain2 : Gain  Gain=1/g
  Gain3 : Gain  Gain=Estimator.gyroAngleUpdateAccWeight
  Gain4 : Gain  Gain=1-Estimator.gyroAngleUpdateAccWeight
  Mux : Mux  Inputs=2
  FAULT_Mux : F_Line_block/Subsystem
  FAULT_Mux_2 : F_Line_block/Subsystem
  Sum : Sum  Inputs=|++
  FAULT_Sum : F_Line_block/Subsystem
  FAULT_Sum_2 : F_Line_block/Subsystem
  Sum1 : Sum  Inputs=|++
  FAULT_Sum1 : F_Line_block/Subsystem
  FAULT_Sum1_2 : F_Line_block/Subsystem
  Terminator1 : Terminator
  FAULT_Terminator1 : F_Line_block/Subsystem
  Trigonometric Function : Trigonometry  Operator=atan
  FAULT_Trigonometric Function : F_Line_block/Subsystem
  Trigonometric Function1 : Trigonometry  Operator=asin
  FAULT_Trigonometric Function1 : F_Line_block/Subsystem
  pitch,roll : Outport
  FAULT_pitch,roll : F_Line_block/Subsystem
  wires:
  accel/1 -> FAULT_Demux/1
  FAULT_Demux/1 -> Demux/1
  Demux/2 -> FAULT_Divide/1
  FAULT_Divide/1 -> Divide/1
  Demux/3 -> FAULT_Divide_2/1
  FAULT_Divide_2/1 -> Divide/2
  Divide/1 -> FAULT_Trigonometric Function/1
  FAULT_Trigonometric Function/1 -> Trigonometric Function/1
  Gain/1 -> FAULT_Sum/1
  FAULT_Sum/1 -> Sum/1
  Trigonometric Function/1 -> FAULT_Gain1/1
  FAULT_Gain1/1 -> Gain1/1
  Mux/1 -> FAULT_pitch,roll/1
  FAULT_pitch,roll/1 -> pitch,roll/1
  Gain2/1 -> FAULT_Trigonometric Function1/1
  FAULT_Trigonometric Function1/1 -> Trigonometric Function1/1
  Trigonometric Function1/1 -> FAULT_Gain3/1
  FAULT_Gain3/1 -> Gain3/1
  Gain4/1 -> FAULT_Sum1/1
  FAULT_Sum1/1 -> Sum1/1
  Gain3/1 -> FAULT_Sum1_2/1
  FAULT_Sum1_2/1 -> Sum1/2
  Sum1/1 -> FAULT_Mux/1
  FAULT_Mux/1 -> Mux/1
  Sum/1 -> FAULT_Mux_2/1
  FAULT_Mux_2/1 -> Mux/2
  rpy/1 -> FAULT_Demux1/1
  FAULT_Demux1/1 -> Demux1/1
  Demux1/1 -> FAULT_Gain/1
  FAULT_Gain/1 -> Gain/1
  Demux1/2 -> FAULT_Gain4/1
  FAULT_Gain4/1 -> Gain4/1
  Demux/1 -> FAULT_Gain2/1
  FAULT_Gain2/1 -> Gain2/1
  Demux1/3 -> FAULT_Terminator1/1
  FAULT_Terminator1/1 -> Terminator1/1
  Gain1/1 -> FAULT_Sum_2/1
  FAULT_Sum_2/1 -> Sum/2

== system state_estimator/State Estimator/Complementary Filter/If Action Subsystem1 ==
  rpy : Inport
  yawVis : Inport  Port=2
  Action Port : ActionPort
  FAULT_Action Port : F_Line_block/Subsystem
  Gain : Gain  Gain=1-Estimator.gyroAngleUpdateVisWeight
  FAULT_Gain : F_Line_block/Subsystem
  Gain1 : Gain  Gain=Estimator.gyroAngleUpdateVisWeight
  FAULT_Gain1 : F_Line_block/Subsystem
  Selector4 : Selector  InputPortWidth=3  IndexOptions=Index vector (dialog)  Indices=[3]  OutputSizes=1
  Sum : Sum  Inputs=|++
  FAULT_Sum : F_Line_block/Subsystem
  FAULT_Sum_2 : F_Line_block/Subsystem
  yaw : Outport
  FAULT_yaw : F_Line_block/Subsystem
  wires:
  rpy/1 -> Selector4/1
  Selector4/1 -> FAULT_Gain/1
  FAULT_Gain/1 -> Gain/1
  yawVis/1 -> FAULT_Gain1/1
  FAULT_Gain1/1 -> Gain1/1
  Gain/1 -> FAULT_Sum/1
  FAULT_Sum/1 -> Sum/1
  Gain1/1 -> FAULT_Sum_2/1
  FAULT_Sum_2/1 -> Sum/2
  Sum/1 -> FAULT_yaw/1
  FAULT_yaw/1 -> yaw/1

== system state_estimator/State Estimator/Complementary Filter/If Action Subsystem2 ==
  prin : Inport
  Action Port : ActionPort
  FAULT_Action Port : F_Line_block/Subsystem
  prout : Outport
  FAULT_prout : F_Line_block/Subsystem
  wires:
  prin/1 -> FAULT_prout/1
  FAULT_prout/1 -> prout/1

== system state_estimator/State Estimator/Complementary Filter/If Action Subsystem3 ==
  yawin : Inport
  Action Port : ActionPort
  FAULT_Action Port : F_Line_block/Subsystem
  yout : Outport
  FAULT_yout : F_Line_block/Subsystem
  wires:
  yawin/1 -> FAULT_yout/1
  FAULT_yout/1 -> yout/1

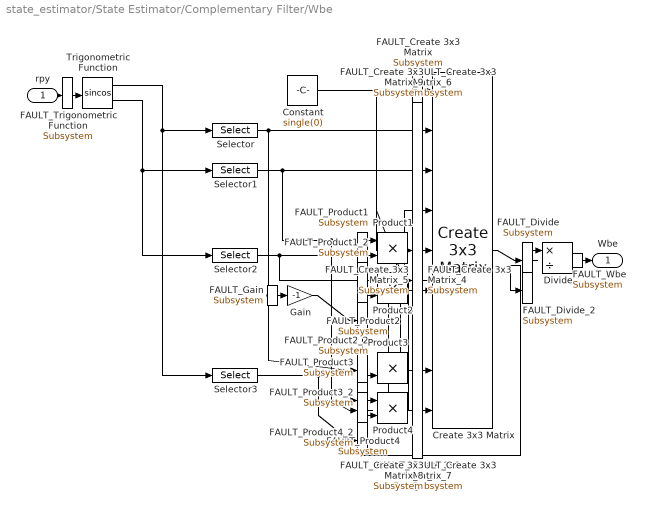
== system state_estimator/State Estimator/Complementary Filter/Wbe ==
  rpy : Inport  OutDataTypeStr=single
  Constant : Constant  Value=single(0)
  Create 3x3 Matrix : sharedutil/Create 3x3 Matrix  aMode=aMode
  FAULT_Create 3x3 Matrix : F_Line_block/Subsystem
  FAULT_Create 3x3 Matrix_{2..9} (8 alike) : F_Line_block/Subsystem
  Divide : Product  Inputs=*/
  FAULT_Divide : F_Line_block/Subsystem
  FAULT_Divide_2 : F_Line_block/Subsystem
  Gain : Gain  Gain=-1
  FAULT_Gain : F_Line_block/Subsystem
  Product{1..4} (4 alike) : Product
  FAULT_Product{1..4} (4 alike) : F_Line_block/Subsystem
  FAULT_Product1_2 : F_Line_block/Subsystem
  FAULT_Product2_2 : F_Line_block/Subsystem
  FAULT_Product3_2 : F_Line_block/Subsystem
  FAULT_Product4_2 : F_Line_block/Subsystem
  Selector : Selector  InputPortWidth=3  IndexOptions=Index vector (dialog)  Indices=[1]  OutputSizes=1
  Selector1 : Selector  InputPortWidth=3  IndexOptions=Index vector (dialog)  Indices=[1]  OutputSizes=1
  Selector2 : Selector  InputPortWidth=3  IndexOptions=Index vector (dialog)  Indices=[2]  OutputSizes=1
  Selector3 : Selector  InputPortWidth=3  IndexOptions=Index vector (dialog)  Indices=[2]  OutputSizes=1
  Trigonometric Function : Trigonometry  Operator=sincos
  FAULT_Trigonometric Function : F_Line_block/Subsystem
  Wbe : Outport
  FAULT_Wbe : F_Line_block/Subsystem
  wires:
  Create 3x3 Matrix/1 -> FAULT_Divide/1
  FAULT_Divide/1 -> Divide/1
  Product3/1 -> FAULT_Create 3x3 Matrix_8/1
  FAULT_Create 3x3 Matrix_8/1 -> Create 3x3 Matrix/8
  Trigonometric Function/2 -> Selector1/1, Selector2/1
  Selector3/1 -> FAULT_Product4_2/1, FAULT_Product3_2/1
  FAULT_Product4_2/1 -> Product4/2
  FAULT_Product3_2/1 -> Product3/2
  Selector1/1 -> FAULT_Product4/1, Product1/1, Create 3x3 Matrix/3
  Trigonometric Function/1 -> Selector3/1, Selector/1
  Product1/1 -> FAULT_Create 3x3 Matrix_5/1
  FAULT_Product4/1 -> Product4/1
  FAULT_Create 3x3 Matrix_5/1 -> Create 3x3 Matrix/5
  Product2/1 -> FAULT_Create 3x3 Matrix_6/1
  FAULT_Create 3x3 Matrix_6/1 -> Create 3x3 Matrix/6
  Selector2/1 -> FAULT_Divide_2/1, FAULT_Create 3x3 Matrix_7/1, Product2/1, Product1/2
  Gain/1 -> FAULT_Product2_2/1
  FAULT_Product2_2/1 -> Product2/2
  Product4/1 -> FAULT_Create 3x3 Matrix_9/1
  FAULT_Create 3x3 Matrix_9/1 -> Create 3x3 Matrix/9
  Constant/1 -> FAULT_Create 3x3 Matrix_4/1, FAULT_Create 3x3 Matrix/1
  FAULT_Create 3x3 Matrix_4/1 -> Create 3x3 Matrix/4
  FAULT_Create 3x3 Matrix/1 -> Create 3x3 Matrix/1
  Divide/1 -> FAULT_Wbe/1
  FAULT_Wbe/1 -> Wbe/1
  rpy/1 -> FAULT_Trigonometric Function/1
  FAULT_Trigonometric Function/1 -> Trigonometric Function/1
  Selector/1 -> FAULT_Product3/1, Gain/1, Create 3x3 Matrix/2

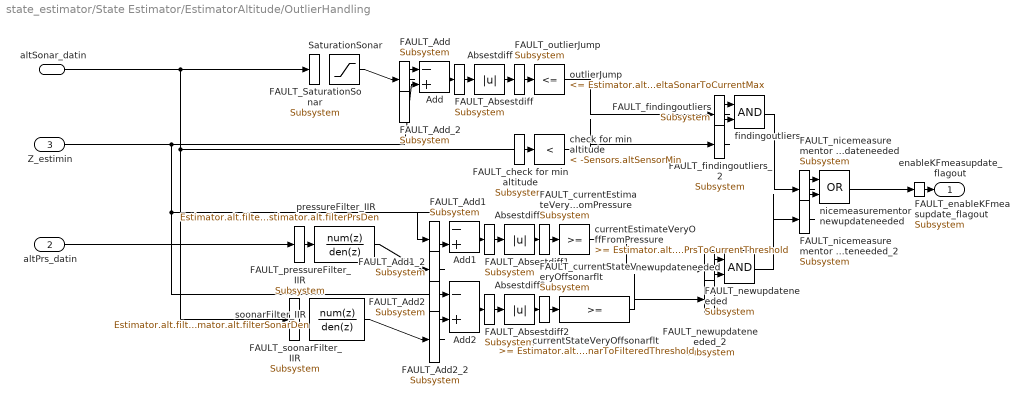
== system state_estimator/State Estimator/EstimatorAltitude/OutlierHandling ==
  altSonar_datin : Inport
  altPrs_datin : Inport  Port=2
  Z_estimin : Inport  Port=3
  Absestdiff : Abs
  FAULT_Absestdiff : F_Line_block/Subsystem
  Absestdiff1 : Abs
  FAULT_Absestdiff1 : F_Line_block/Subsystem
  Absestdiff2 : Abs
  FAULT_Absestdiff2 : F_Line_block/Subsystem
  Add : Sum  Inputs=-+
  FAULT_Add : F_Line_block/Subsystem
  FAULT_Add_2 : F_Line_block/Subsystem
  Add1 : Sum  Inputs=-+
  FAULT_Add1 : F_Line_block/Subsystem
  FAULT_Add1_2 : F_Line_block/Subsystem
  Add2 : Sum  Inputs=-+
  FAULT_Add2 : F_Line_block/Subsystem
  FAULT_Add2_2 : F_Line_block/Subsystem
  SaturationSonar : Saturate  UpperLimit=-Sensors.altSensorMin  LowerLimit=-inf
  FAULT_SaturationSonar : F_Line_block/Subsystem
  check for min altitude : simulink/Logic and Bit Operations/Compare To Constant  relop=<  const=-Sensors.altSensorMin  OutDataTypeStr=boolean
  FAULT_check for min altitude : F_Line_block/Subsystem
  currentEstimateVeryOffFromPressure : simulink/Logic and Bit Operations/Compare To Constant  relop=>=  const=Estimator.alt.deltaPrsToCurrentThreshold  OutDataTypeStr=boolean
  FAULT_currentEstimateVeryOffFromPressure : F_Line_block/Subsystem
  currentStateVeryOffsonarflt : simulink/Logic and Bit Operations/Compare To Constant  relop=>=  const=Estimator.alt.deltaSonarToFilteredThreshold  OutDataTypeStr=boolean
  FAULT_currentStateVeryOffsonarflt : F_Line_block/Subsystem
  findingoutliers : Logic  AllPortsSameDT=off  OutDataTypeStr=boolean
  FAULT_findingoutliers : F_Line_block/Subsystem
  FAULT_findingoutliers_2 : F_Line_block/Subsystem
  newupdateneeded : Logic  AllPortsSameDT=off  OutDataTypeStr=boolean
  FAULT_newupdateneeded : F_Line_block/Subsystem
  FAULT_newupdateneeded_2 : F_Line_block/Subsystem
  nicemeasurementor newupdateneeded : Logic  Operator=OR  AllPortsSameDT=off  OutDataTypeStr=boolean
  FAULT_nicemeasurementor newupdateneeded : F_Line_block/Subsystem
  FAULT_nicemeasurementor newupdateneeded_2 : F_Line_block/Subsystem
  outlierJump : simulink/Logic and Bit Operations/Compare To Constant  relop=<=  const=Estimator.alt.deltaSonarToCurrentMax  OutDataTypeStr=boolean
  FAULT_outlierJump : F_Line_block/Subsystem
  pressureFilter_IIR : DiscreteFilter  Numerator=Estimator.alt.filterPrsNum  Denominator=Estimator.alt.filterPrsDen
  FAULT_pressureFilter_IIR : F_Line_block/Subsystem
  soonarFilter_IIR : DiscreteFilter  Numerator=Estimator.alt.filterSonarNum  Denominator=Estimator.alt.filterSonarDen
  FAULT_soonarFilter_IIR : F_Line_block/Subsystem
  enableKFmeasupdate_flagout : Outport
  FAULT_enableKFmeasupdate_flagout : F_Line_block/Subsystem
  wires:
  Add1/1 -> FAULT_Absestdiff1/1
  FAULT_Absestdiff1/1 -> Absestdiff1/1
  nicemeasurementor newupdateneeded/1 -> FAULT_enableKFmeasupdate_flagout/1
  FAULT_enableKFmeasupdate_flagout/1 -> enableKFmeasupdate_flagout/1
  findingoutliers/1 -> FAULT_nicemeasurementor newupdateneeded/1
  FAULT_nicemeasurementor newupdateneeded/1 -> nicemeasurementor newupdateneeded/1
  check for min altitude/1 -> FAULT_findingoutliers_2/1
  FAULT_findingoutliers_2/1 -> findingoutliers/2
  outlierJump/1 -> FAULT_findingoutliers/1
  FAULT_findingoutliers/1 -> findingoutliers/1
  SaturationSonar/1 -> FAULT_Add/1
  FAULT_Add/1 -> Add/1
  Absestdiff/1 -> FAULT_outlierJump/1
  FAULT_outlierJump/1 -> outlierJump/1
  Add/1 -> FAULT_Absestdiff/1
  FAULT_Absestdiff/1 -> Absestdiff/1
  newupdateneeded/1 -> FAULT_nicemeasurementor newupdateneeded_2/1
  FAULT_nicemeasurementor newupdateneeded_2/1 -> nicemeasurementor newupdateneeded/2
  Absestdiff2/1 -> FAULT_currentStateVeryOffsonarflt/1
  FAULT_currentStateVeryOffsonarflt/1 -> currentStateVeryOffsonarflt/1
  altSonar_datin/1 -> FAULT_SaturationSonar/1, FAULT_soonarFilter_IIR/1, check for min altitude/1
  currentEstimateVeryOffFromPressure/1 -> FAULT_newupdateneeded/1
  FAULT_newupdateneeded/1 -> newupdateneeded/1
  Z_estimin/1 -> FAULT_Add1/1, Add2/1, Add/2
  Add2/1 -> FAULT_Absestdiff2/1
  FAULT_Absestdiff2/1 -> Absestdiff2/1
  currentStateVeryOffsonarflt/1 -> FAULT_newupdateneeded_2/1
  FAULT_newupdateneeded_2/1 -> newupdateneeded/2
  pressureFilter_IIR/1 -> FAULT_Add1_2/1
  FAULT_Add1_2/1 -> Add1/2
  altPrs_datin/1 -> FAULT_pressureFilter_IIR/1
  FAULT_pressureFilter_IIR/1 -> pressureFilter_IIR/1
  soonarFilter_IIR/1 -> FAULT_Add2_2/1
  FAULT_Add2_2/1 -> Add2/2
  Absestdiff1/1 -> FAULT_currentEstimateVeryOffFromPressure/1
  FAULT_currentEstimateVeryOffFromPressure/1 -> currentEstimateVeryOffFromPressure/1

== system state_estimator/State Estimator/EstimatorXYPosition/EstimatorVelocity ==
  opticalFlow_datin : Inport
  Z_estimin : Inport  Port=2  SampleTime=Ts
  sensorIMU_datin : Inport  Port=3
  orient_estimin : Inport  Port=4
  AccelerationHandling : Subsystem
  DataHandling : Subsystem
  Delay : Delay  DelayLength=1  InitialCondition=0
  FAULT_Delay : F_Line_block/Subsystem
  KalmanFilter_dxdy : ctrlSharedLib/Kalman Filter  TimeDomain=Discrete-Time  UseCurrentEstimator=on  ModelSource=Individual A, B, C, D matrices  ModelSourceVariable=ss(0.95,1,1,0,1)  A=eye(2)  B=Ts*eye(2)  C=eye(2)  D=0  NumberOfStates=1  NumberOfInputs=1  NumberOfOutputs=1  InitialEstimateSource=Dialog  X0=0  P0=10  UseK=off  UseGH=on  NumberOfProcessNoiseInputs=1  G=Estimator.pos.kfVelo.G  TimeInvariantG=on  H=Estimator.pos.kfVelo.H  TimeInvariantH=on  Q=Estimator.pos.kfVelo.Q  TimeInvariantQ=on  R=Estimator.pos.kfVelo.R  TimeInvariantR=on  N=Estimator.pos.kfVelo.N  TimeInvariantN=on  AddInputPort=on  AddEnablePort=on  OutputEstimatedY=off  OutputP=off  Ts=-1
      settings: SourceProductBaseCode=CT
  FAULT_KalmanFilter_dxdy : F_Line_block/Subsystem
  FAULT_KalmanFilter_dxdy_2 : F_Line_block/Subsystem
  FAULT_KalmanFilter_dxdy_3 : F_Line_block/Subsystem
  Select dxy : Selector  InputPortWidth=3  IndexOptions=Index vector (dialog)  Indices=[1 2]  OutputSizes=1
  opticalFlowToVelocity_gain : Gain  Gain=Estimator.pos.opticalFlowToVelocityGain
  FAULT_opticalFlowToVelocity_gain : F_Line_block/Subsystem
  dxy_estimout : Outport
  FAULT_dxy_estimout : F_Line_block/Subsystem
  wires:
  Delay/1 -> DataHandling/5(dxyOF_datin)
  Z_estimin/1 -> DataHandling/1(Z_estimin), AccelerationHandling/4(Z_estimin)
  KalmanFilter_dxdy/1 -> FAULT_dxy_estimout/1, FAULT_Delay/1
  ?FAULT_Demux1/1 -> ?Demux1/1
  ?FAULT_IIRgyroz/1 -> ?IIRgyroz/1
  FAULT_dxy_estimout/1 -> dxy_estimout/1
  FAULT_Delay/1 -> Delay/1
  opticalFlowToVelocity_gain/1 -> Select dxy/1
  opticalFlow_datin/1 -> FAULT_opticalFlowToVelocity_gain/1
  FAULT_opticalFlowToVelocity_gain/1 -> opticalFlowToVelocity_gain/1
  sensorIMU_datin/1 -> AccelerationHandling/2(sensorIMU_datin), DataHandling/3(sensorIMU_datin)
  orient_estimin/1 -> AccelerationHandling/3(orient_estimin), DataHandling/2(orient_estimin)
  Select dxy/1 -> FAULT_KalmanFilter_dxdy_2/1, AccelerationHandling/1(dxy_estimin), DataHandling/4(dxy_estimin)
  AccelerationHandling/1(acceleration_world) -> FAULT_KalmanFilter_dxdy/1
  FAULT_KalmanFilter_dxdy/1 -> KalmanFilter_dxdy/1
  DataHandling/1(enable_flag) -> FAULT_KalmanFilter_dxdy_3/1
  FAULT_KalmanFilter_dxdy_3/1 -> KalmanFilter_dxdy/3

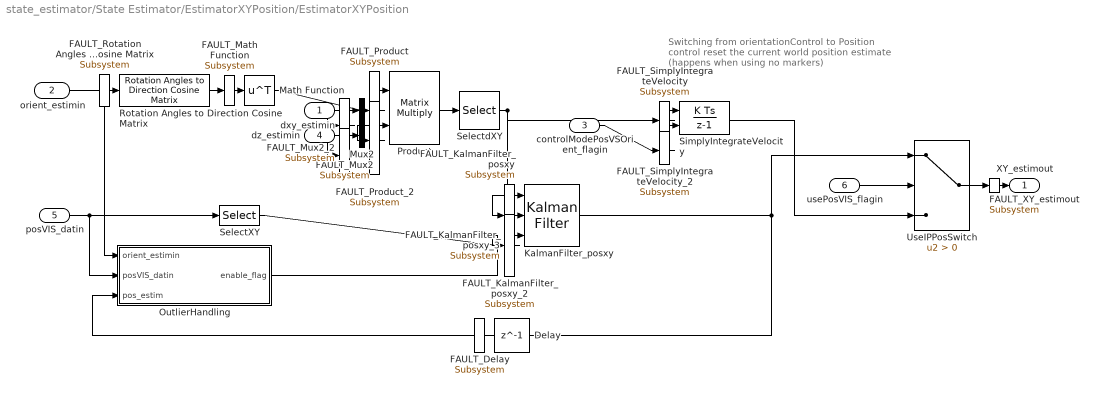
== system state_estimator/State Estimator/EstimatorXYPosition/EstimatorXYPosition ==
  note: Switching from orientationControl to Position
      | control reset the current world position estimate
      | (happens when using no markers)
  dxy_estimin : Inport
  orient_estimin : Inport  Port=2  SampleTime=Ts
  controlModePosVSOrient_flagin : Inport  Port=3
  dz_estimin : Inport  Port=4
  posVIS_datin : Inport  Port=5
  usePosVIS_flagin : Inport  Port=6
  Delay : Delay  DelayLength=1  InitialCondition=0
  FAULT_Delay : F_Line_block/Subsystem
  KalmanFilter_posxy : ctrlSharedLib/Kalman Filter  TimeDomain=Discrete-Time  UseCurrentEstimator=on  ModelSource=Individual A, B, C, D matrices  ModelSourceVariable=ss(0.95,1,1,0,1)  A=eye(2)  B=Ts*eye(2)  C=eye(2)  D=0  NumberOfStates=1  NumberOfInputs=1  NumberOfOutputs=1  InitialEstimateSource=Dialog  X0=[.1 0]  P0=10  UseK=off  UseGH=on  NumberOfProcessNoiseInputs=1  G=Estimator.pos.kfPos.G  TimeInvariantG=on  H=Estimator.pos.kfPos.H  TimeInvariantH=on  Q=Estimator.pos.kfPos.Q  TimeInvariantQ=on  R=Estimator.pos.kfPos.R  TimeInvariantR=on  N=Estimator.pos.kfPos.N  TimeInvariantN=on  AddInputPort=on  AddEnablePort=on  OutputEstimatedY=off  OutputP=off  Ts=-1
      settings: SourceProductBaseCode=CT
  FAULT_KalmanFilter_posxy : F_Line_block/Subsystem
  FAULT_KalmanFilter_posxy_2 : F_Line_block/Subsystem
  FAULT_KalmanFilter_posxy_3 : F_Line_block/Subsystem
  Math Function : Math  Operator=transpose  SaturateOnIntegerOverflow=on
  FAULT_Math Function : F_Line_block/Subsystem
  Mux2 : Mux  Inputs=2
  FAULT_Mux2 : F_Line_block/Subsystem
  FAULT_Mux2_2 : F_Line_block/Subsystem
  OutlierHandling : Subsystem
  Product : Product  Multiplication=Matrix(*)
  FAULT_Product : F_Line_block/Subsystem
  FAULT_Product_2 : F_Line_block/Subsystem
  Rotation Angles to Direction Cosine Matrix : sharedtransform/Rotation Angles to Direction Cosine Matrix  rotationOrder=ZYX  aMode=aMode
      settings: SourceProductBaseCode=AE
  FAULT_Rotation Angles to Direction Cosine Matrix : F_Line_block/Subsystem
  SelectXY : Selector  InputPortWidth=4  IndexOptions=Index vector (dialog)  Indices=[1 2]  OutputSizes=1
  SelectdXY : Selector  InputPortWidth=3  IndexOptions=Index vector (dialog)  Indices=[1 2]  OutputSizes=1
  SimplyIntegrateVelocity : DiscreteIntegrator  ExternalReset=rising  SampleTime=Ts  ICPrevOutput=DiscIntNeverNeededParam  ICPrevScaledInput=DiscIntNeverNeededParam
  FAULT_SimplyIntegrateVelocity : F_Line_block/Subsystem
  FAULT_SimplyIntegrateVelocity_2 : F_Line_block/Subsystem
  UseIPPosSwitch : Switch  Criteria=u2 > Threshold
  XY_estimout : Outport
  FAULT_XY_estimout : F_Line_block/Subsystem
  wires:
  Delay/1 -> OutlierHandling/3(pos_estim)
  usePosVIS_flagin/1 -> UseIPPosSwitch/2
  UseIPPosSwitch/1 -> FAULT_XY_estimout/1
  FAULT_XY_estimout/1 -> XY_estimout/1
  controlModePosVSOrient_flagin/1 -> FAULT_SimplyIntegrateVelocity_2/1
  FAULT_SimplyIntegrateVelocity_2/1 -> SimplyIntegrateVelocity/2
  KalmanFilter_posxy/1 -> FAULT_Delay/1, UseIPPosSwitch/1
  FAULT_Delay/1 -> Delay/1
  ?FAULT_IIRgyroz/1 -> ?IIRgyroz/1
  posVIS_datin/1 -> OutlierHandling/2(posVIS_datin), SelectXY/1
  Product/1 -> SelectdXY/1
  Mux2/1 -> FAULT_Product_2/1
  FAULT_Delay/1 -> Delay/1
  ?FAULT_IIRgyroz/1 -> ?IIRgyroz/1
  ?FAULT_Sqrt/1 -> ?Sqrt/1
  FAULT_Product_2/1 -> Product/2
  dz_estimin/1 -> FAULT_Mux2_2/1
  FAULT_Mux2_2/1 -> Mux2/2
  SimplyIntegrateVelocity/1 -> UseIPPosSwitch/3
  dxy_estimin/1 -> FAULT_Mux2/1
  FAULT_Mux2/1 -> Mux2/1
  orient_estimin/1 -> FAULT_Rotation Angles to Direction Cosine Matrix/1, OutlierHandling/1(orient_estimin)
  FAULT_Rotation Angles to Direction Cosine Matrix/1 -> Rotation Angles to Direction Cosine Matrix/1
  ?FAULT_IIRgyroz/1 -> ?IIRgyroz/1
  Rotation Angles to Direction Cosine Matrix/1 -> FAULT_Math Function/1
  FAULT_Math Function/1 -> Math Function/1
  SelectXY/1 -> FAULT_KalmanFilter_posxy_2/1
  FAULT_KalmanFilter_posxy_2/1 -> KalmanFilter_posxy/2
  OutlierHandling/1(enable_flag) -> FAULT_KalmanFilter_posxy_3/1
  FAULT_KalmanFilter_posxy_3/1 -> KalmanFilter_posxy/3
  SelectdXY/1 -> FAULT_SimplyIntegrateVelocity/1, FAULT_KalmanFilter_posxy/1
  FAULT_SimplyIntegrateVelocity/1 -> SimplyIntegrateVelocity/1
  FAULT_KalmanFilter_posxy/1 -> KalmanFilter_posxy/1
  Math Function/1 -> FAULT_Product/1
  FAULT_Product/1 -> Product/1
